simulink model "8Bit_MUX"  (R2019b)
settings: Solver=VariableStepAuto  StartTime=0.0  StopTime=10.0  RelTol=1e-3
libraries: hdlsllib x49
settings Model: Creator=cohen  LastModifiedBy=cohen

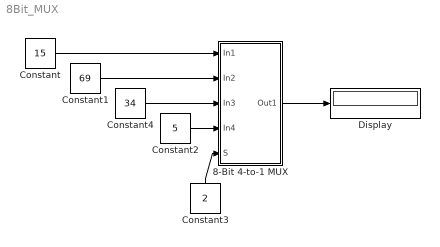
== system 8Bit_MUX ==
  8-Bit 4-to-1 MUX : Subsystem
  Constant : Constant  Value=15  OutDataTypeStr=uint8
  Constant1 : Constant  Value=69  OutDataTypeStr=uint8
  Constant2 : Constant  Value=5  OutDataTypeStr=uint8
  Constant3 : Constant  Value=2  OutDataTypeStr=uint8
  Constant4 : Constant  Value=34  OutDataTypeStr=uint8
  Display : Display
  wires:
  8-Bit 4-to-1 MUX/1(Out1) -> Display/1
  Constant/1 -> 8-Bit 4-to-1 MUX/1(In1)
  Constant1/1 -> 8-Bit 4-to-1 MUX/2(In2)
  Constant4/1 -> 8-Bit 4-to-1 MUX/3(In3)
  Constant2/1 -> 8-Bit 4-to-1 MUX/4(In4)
  Constant3/1 -> 8-Bit 4-to-1 MUX/5(S)

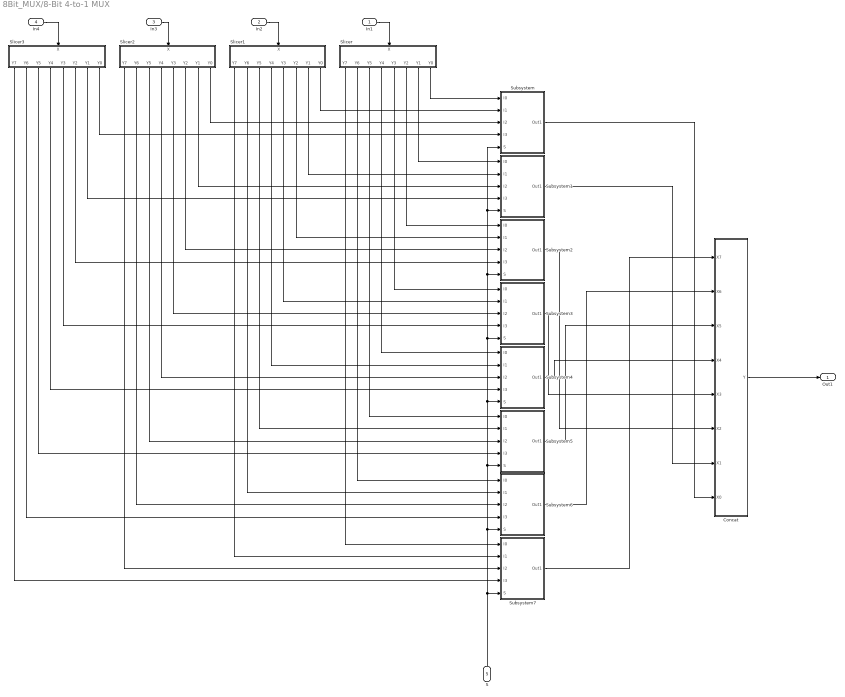
== system 8Bit_MUX/8-Bit 4-to-1 MUX ==
  In1 : Inport  OutDataTypeStr=uint8
  In2 : Inport  Port=2  OutDataTypeStr=uint8
  In3 : Inport  Port=3  OutDataTypeStr=uint8
  In4 : Inport  Port=4  OutDataTypeStr=uint8
  S : Inport  Port=5  OutDataTypeStr=uint8
  Concat : Subsystem
  Slicer : Subsystem
  Slicer1 : Subsystem
  Slicer2 : Subsystem
  Slicer3 : Subsystem
  Subsystem : Subsystem
  Subsystem1 : Subsystem
  Subsystem2 : Subsystem
  Subsystem3 : Subsystem
  Subsystem4 : Subsystem
  Subsystem5 : Subsystem
  Subsystem6 : Subsystem
  Subsystem7 : Subsystem
  Out1 : Outport  OutDataTypeStr=uint8
  wires:
  Slicer1/8(Y0) -> Subsystem/2(I1)
  Subsystem3/1(Out1) -> Concat/5(X3)
  Slicer/6(Y2) -> Subsystem2/1(I0)
  Slicer2/7(Y1) -> Subsystem1/3(I2)
  Subsystem2/1(Out1) -> Concat/6(X2)
  Concat/1(Y) -> Out1/1
  S/1 -> Subsystem7/5(S), Subsystem4/5(S), Subsystem1/5(S), Subsystem/5(S), Subsystem2/5(S), Subsystem3/5(S), Subsystem5/5(S), Subsystem6/5(S)
  Subsystem6/1(Out1) -> Concat/2(X6)
  Slicer2/3(Y5) -> Subsystem5/3(I2)
  Slicer3/4(Y4) -> Subsystem4/4(I3)
  Slicer2/2(Y6) -> Subsystem6/3(I2)
  Slicer/2(Y6) -> Subsystem6/1(I0)
  In2/1 -> Slicer1/1(X)
  Slicer2/1(Y7) -> Subsystem7/3(I2)
  Slicer3/7(Y1) -> Subsystem1/4(I3)
  Slicer/5(Y3) -> Subsystem3/1(I0)
  Slicer3/6(Y2) -> Subsystem2/4(I3)
  In1/1 -> Slicer/1(X)
  Slicer1/1(Y7) -> Subsystem7/2(I1)
  In3/1 -> Slicer2/1(X)
  Slicer/8(Y0) -> Subsystem/1(I0)
  Slicer1/4(Y4) -> Subsystem4/2(I1)
  Slicer2/4(Y4) -> Subsystem4/3(I2)
  Slicer1/3(Y5) -> Subsystem5/2(I1)
  Slicer3/5(Y3) -> Subsystem3/4(I3)
  Slicer/4(Y4) -> Subsystem4/1(I0)
  Slicer2/8(Y0) -> Subsystem/3(I2)
  Slicer1/5(Y3) -> Subsystem3/2(I1)
  Slicer1/7(Y1) -> Subsystem1/2(I1)
  Subsystem7/1(Out1) -> Concat/1(X7)
  Slicer1/6(Y2) -> Subsystem2/2(I1)
  Subsystem/1(Out1) -> Concat/8(X0)
  Subsystem4/1(Out1) -> Concat/4(X4)
  Subsystem5/1(Out1) -> Concat/3(X5)
  Slicer1/2(Y6) -> Subsystem6/2(I1)
  Slicer3/8(Y0) -> Subsystem/4(I3)
  Slicer2/6(Y2) -> Subsystem2/3(I2)
  Slicer/3(Y5) -> Subsystem5/1(I0)
  Slicer3/3(Y5) -> Subsystem5/4(I3)
  Slicer3/2(Y6) -> Subsystem6/4(I3)
  Slicer3/1(Y7) -> Subsystem7/4(I3)
  Slicer2/5(Y3) -> Subsystem3/3(I2)
  In4/1 -> Slicer3/1(X)
  Subsystem1/1(Out1) -> Concat/7(X1)
  Slicer/1(Y7) -> Subsystem7/1(I0)
  Slicer/7(Y1) -> Subsystem1/1(I0)

== system 8Bit_MUX/8-Bit 4-to-1 MUX/Concat ==
  X7 : Inport  OutDataTypeStr=boolean  SampleTime=1
  X6 : Inport  Port=2  OutDataTypeStr=boolean  SampleTime=1
  X5 : Inport  Port=3  OutDataTypeStr=boolean  SampleTime=1
  X4 : Inport  Port=4  OutDataTypeStr=boolean  SampleTime=1
  X3 : Inport  Port=5  OutDataTypeStr=boolean  SampleTime=1
  X2 : Inport  Port=6  OutDataTypeStr=boolean  SampleTime=1
  X1 : Inport  Port=7  OutDataTypeStr=boolean  SampleTime=1
  X0 : Inport  Port=8  OutDataTypeStr=boolean  SampleTime=1
  Bit Concat : hdlsllib/Logic and Bit Operations/Bit Concat  numInputs=8
      settings: SourceProductName=Simulink
  Y : Outport  SampleTime=1
  wires:
  X6/1 -> Bit Concat/2
  X2/1 -> Bit Concat/6
  X7/1 -> Bit Concat/1
  X0/1 -> Bit Concat/8
  Bit Concat/1 -> Y/1
  X3/1 -> Bit Concat/5
  X1/1 -> Bit Concat/7
  X5/1 -> Bit Concat/3
  X4/1 -> Bit Concat/4

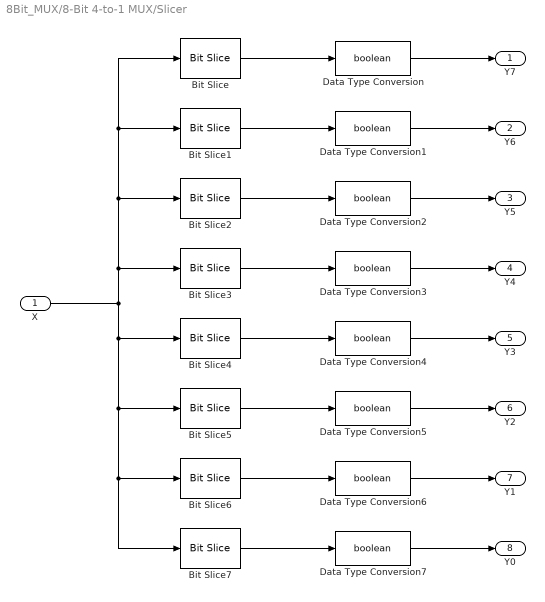
== system 8Bit_MUX/8-Bit 4-to-1 MUX/Slicer ==
  X : Inport  OutDataTypeStr=uint8  SampleTime=1
  Bit Slice : hdlsllib/Logic and Bit Operations/Bit Slice  lidx=7  ridx=7
      settings: SourceProductName=Simulink  SourceProductBaseCode=SL
  Bit Slice1 : hdlsllib/Logic and Bit Operations/Bit Slice  lidx=6  ridx=6
      settings: SourceProductName=Simulink  SourceProductBaseCode=SL
  Bit Slice2 : hdlsllib/Logic and Bit Operations/Bit Slice  lidx=5  ridx=5
      settings: SourceProductName=Simulink  SourceProductBaseCode=SL
  Bit Slice3 : hdlsllib/Logic and Bit Operations/Bit Slice  lidx=4  ridx=4
      settings: SourceProductName=Simulink  SourceProductBaseCode=SL
  Bit Slice4 : hdlsllib/Logic and Bit Operations/Bit Slice  lidx=3  ridx=3
      settings: SourceProductName=Simulink  SourceProductBaseCode=SL
  Bit Slice5 : hdlsllib/Logic and Bit Operations/Bit Slice  lidx=2  ridx=2
      settings: SourceProductName=Simulink  SourceProductBaseCode=SL
  Bit Slice6 : hdlsllib/Logic and Bit Operations/Bit Slice  lidx=1  ridx=1
      settings: SourceProductName=Simulink  SourceProductBaseCode=SL
  Bit Slice7 : hdlsllib/Logic and Bit Operations/Bit Slice  lidx=0  ridx=0
      settings: SourceProductName=Simulink  SourceProductBaseCode=SL
  Data Type Conversion{,1..7} (8 alike) : DataTypeConversion  OutDataTypeStr=boolean
  Y7 : Outport  OutDataTypeStr=boolean  SampleTime=1
  Y6 : Outport  Port=2  OutDataTypeStr=boolean  SampleTime=1
  Y5 : Outport  Port=3  OutDataTypeStr=boolean  SampleTime=1
  Y4 : Outport  Port=4  OutDataTypeStr=boolean
  Y3 : Outport  Port=5  OutDataTypeStr=boolean  SampleTime=1
  Y2 : Outport  Port=6  OutDataTypeStr=boolean  SampleTime=1
  Y1 : Outport  Port=7  OutDataTypeStr=boolean  SampleTime=1
  Y0 : Outport  Port=8  OutDataTypeStr=boolean  SampleTime=1
  wires:
  Bit Slice6/1 -> Data Type Conversion6/1
  X/1 -> Bit Slice3/1, Bit Slice2/1, Bit Slice1/1, Bit Slice/1, Bit Slice4/1, Bit Slice5/1, Bit Slice6/1, Bit Slice7/1
  Bit Slice/1 -> Data Type Conversion/1
  Bit Slice7/1 -> Data Type Conversion7/1
  Bit Slice4/1 -> Data Type Conversion4/1
  Bit Slice1/1 -> Data Type Conversion1/1
  Bit Slice3/1 -> Data Type Conversion3/1
  Data Type Conversion1/1 -> Y6/1
  Data Type Conversion7/1 -> Y0/1
  Data Type Conversion5/1 -> Y2/1
  Data Type Conversion3/1 -> Y4/1
  Data Type Conversion4/1 -> Y3/1
  Bit Slice2/1 -> Data Type Conversion2/1
  Bit Slice5/1 -> Data Type Conversion5/1
  Data Type Conversion6/1 -> Y1/1
  Data Type Conversion/1 -> Y7/1
  Data Type Conversion2/1 -> Y5/1

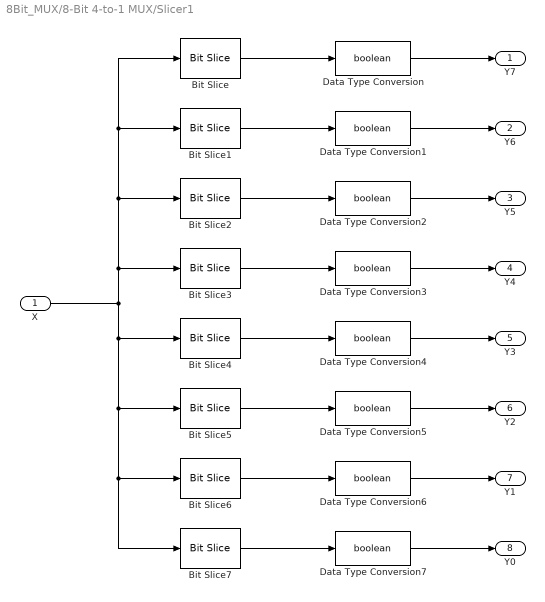
== system 8Bit_MUX/8-Bit 4-to-1 MUX/Slicer1 ==
  X : Inport  OutDataTypeStr=uint8  SampleTime=1
  Bit Slice : hdlsllib/Logic and Bit Operations/Bit Slice  lidx=7  ridx=7
      settings: SourceProductName=Simulink  SourceProductBaseCode=SL
  Bit Slice1 : hdlsllib/Logic and Bit Operations/Bit Slice  lidx=6  ridx=6
      settings: SourceProductName=Simulink  SourceProductBaseCode=SL
  Bit Slice2 : hdlsllib/Logic and Bit Operations/Bit Slice  lidx=5  ridx=5
      settings: SourceProductName=Simulink  SourceProductBaseCode=SL
  Bit Slice3 : hdlsllib/Logic and Bit Operations/Bit Slice  lidx=4  ridx=4
      settings: SourceProductName=Simulink  SourceProductBaseCode=SL
  Bit Slice4 : hdlsllib/Logic and Bit Operations/Bit Slice  lidx=3  ridx=3
      settings: SourceProductName=Simulink  SourceProductBaseCode=SL
  Bit Slice5 : hdlsllib/Logic and Bit Operations/Bit Slice  lidx=2  ridx=2
      settings: SourceProductName=Simulink  SourceProductBaseCode=SL
  Bit Slice6 : hdlsllib/Logic and Bit Operations/Bit Slice  lidx=1  ridx=1
      settings: SourceProductName=Simulink  SourceProductBaseCode=SL
  Bit Slice7 : hdlsllib/Logic and Bit Operations/Bit Slice  lidx=0  ridx=0
      settings: SourceProductName=Simulink  SourceProductBaseCode=SL
  Data Type Conversion{,1..7} (8 alike) : DataTypeConversion  OutDataTypeStr=boolean
  Y7 : Outport  OutDataTypeStr=boolean  SampleTime=1
  Y6 : Outport  Port=2  OutDataTypeStr=boolean  SampleTime=1
  Y5 : Outport  Port=3  OutDataTypeStr=boolean  SampleTime=1
  Y4 : Outport  Port=4  OutDataTypeStr=boolean
  Y3 : Outport  Port=5  OutDataTypeStr=boolean  SampleTime=1
  Y2 : Outport  Port=6  OutDataTypeStr=boolean  SampleTime=1
  Y1 : Outport  Port=7  OutDataTypeStr=boolean  SampleTime=1
  Y0 : Outport  Port=8  OutDataTypeStr=boolean  SampleTime=1
  wires:
  Bit Slice6/1 -> Data Type Conversion6/1
  X/1 -> Bit Slice3/1, Bit Slice2/1, Bit Slice1/1, Bit Slice/1, Bit Slice4/1, Bit Slice5/1, Bit Slice6/1, Bit Slice7/1
  Bit Slice/1 -> Data Type Conversion/1
  Bit Slice7/1 -> Data Type Conversion7/1
  Bit Slice4/1 -> Data Type Conversion4/1
  Bit Slice1/1 -> Data Type Conversion1/1
  Bit Slice3/1 -> Data Type Conversion3/1
  Data Type Conversion1/1 -> Y6/1
  Data Type Conversion7/1 -> Y0/1
  Data Type Conversion5/1 -> Y2/1
  Data Type Conversion3/1 -> Y4/1
  Data Type Conversion4/1 -> Y3/1
  Bit Slice2/1 -> Data Type Conversion2/1
  Bit Slice5/1 -> Data Type Conversion5/1
  Data Type Conversion6/1 -> Y1/1
  Data Type Conversion/1 -> Y7/1
  Data Type Conversion2/1 -> Y5/1

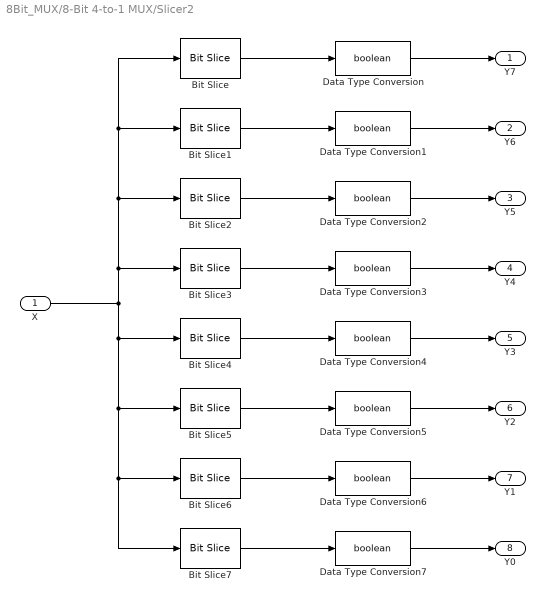
== system 8Bit_MUX/8-Bit 4-to-1 MUX/Slicer2 ==
  X : Inport  OutDataTypeStr=uint8  SampleTime=1
  Bit Slice : hdlsllib/Logic and Bit Operations/Bit Slice  lidx=7  ridx=7
      settings: SourceProductName=Simulink  SourceProductBaseCode=SL
  Bit Slice1 : hdlsllib/Logic and Bit Operations/Bit Slice  lidx=6  ridx=6
      settings: SourceProductName=Simulink  SourceProductBaseCode=SL
  Bit Slice2 : hdlsllib/Logic and Bit Operations/Bit Slice  lidx=5  ridx=5
      settings: SourceProductName=Simulink  SourceProductBaseCode=SL
  Bit Slice3 : hdlsllib/Logic and Bit Operations/Bit Slice  lidx=4  ridx=4
      settings: SourceProductName=Simulink  SourceProductBaseCode=SL
  Bit Slice4 : hdlsllib/Logic and Bit Operations/Bit Slice  lidx=3  ridx=3
      settings: SourceProductName=Simulink  SourceProductBaseCode=SL
  Bit Slice5 : hdlsllib/Logic and Bit Operations/Bit Slice  lidx=2  ridx=2
      settings: SourceProductName=Simulink  SourceProductBaseCode=SL
  Bit Slice6 : hdlsllib/Logic and Bit Operations/Bit Slice  lidx=1  ridx=1
      settings: SourceProductName=Simulink  SourceProductBaseCode=SL
  Bit Slice7 : hdlsllib/Logic and Bit Operations/Bit Slice  lidx=0  ridx=0
      settings: SourceProductName=Simulink  SourceProductBaseCode=SL
  Data Type Conversion{,1..7} (8 alike) : DataTypeConversion  OutDataTypeStr=boolean
  Y7 : Outport  OutDataTypeStr=boolean  SampleTime=1
  Y6 : Outport  Port=2  OutDataTypeStr=boolean  SampleTime=1
  Y5 : Outport  Port=3  OutDataTypeStr=boolean  SampleTime=1
  Y4 : Outport  Port=4  OutDataTypeStr=boolean
  Y3 : Outport  Port=5  OutDataTypeStr=boolean  SampleTime=1
  Y2 : Outport  Port=6  OutDataTypeStr=boolean  SampleTime=1
  Y1 : Outport  Port=7  OutDataTypeStr=boolean  SampleTime=1
  Y0 : Outport  Port=8  OutDataTypeStr=boolean  SampleTime=1
  wires:
  Bit Slice6/1 -> Data Type Conversion6/1
  X/1 -> Bit Slice3/1, Bit Slice2/1, Bit Slice1/1, Bit Slice/1, Bit Slice4/1, Bit Slice5/1, Bit Slice6/1, Bit Slice7/1
  Bit Slice/1 -> Data Type Conversion/1
  Bit Slice7/1 -> Data Type Conversion7/1
  Bit Slice4/1 -> Data Type Conversion4/1
  Bit Slice1/1 -> Data Type Conversion1/1
  Bit Slice3/1 -> Data Type Conversion3/1
  Data Type Conversion1/1 -> Y6/1
  Data Type Conversion7/1 -> Y0/1
  Data Type Conversion5/1 -> Y2/1
  Data Type Conversion3/1 -> Y4/1
  Data Type Conversion4/1 -> Y3/1
  Bit Slice2/1 -> Data Type Conversion2/1
  Bit Slice5/1 -> Data Type Conversion5/1
  Data Type Conversion6/1 -> Y1/1
  Data Type Conversion/1 -> Y7/1
  Data Type Conversion2/1 -> Y5/1

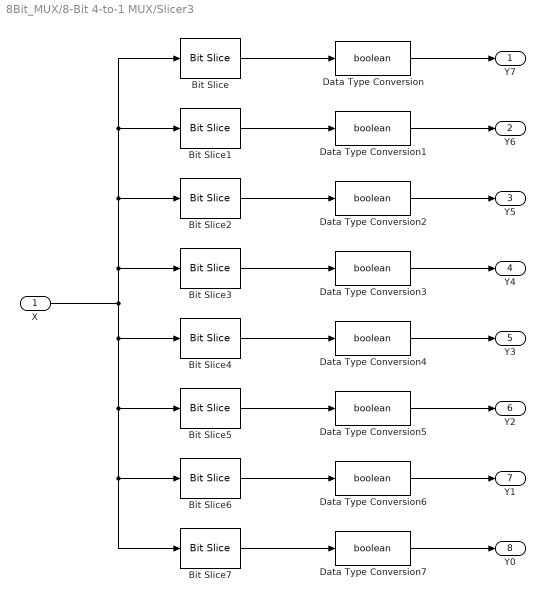
== system 8Bit_MUX/8-Bit 4-to-1 MUX/Slicer3 ==
  X : Inport  OutDataTypeStr=uint8  SampleTime=1
  Bit Slice : hdlsllib/Logic and Bit Operations/Bit Slice  lidx=7  ridx=7
      settings: SourceProductName=Simulink  SourceProductBaseCode=SL
  Bit Slice1 : hdlsllib/Logic and Bit Operations/Bit Slice  lidx=6  ridx=6
      settings: SourceProductName=Simulink  SourceProductBaseCode=SL
  Bit Slice2 : hdlsllib/Logic and Bit Operations/Bit Slice  lidx=5  ridx=5
      settings: SourceProductName=Simulink  SourceProductBaseCode=SL
  Bit Slice3 : hdlsllib/Logic and Bit Operations/Bit Slice  lidx=4  ridx=4
      settings: SourceProductName=Simulink  SourceProductBaseCode=SL
  Bit Slice4 : hdlsllib/Logic and Bit Operations/Bit Slice  lidx=3  ridx=3
      settings: SourceProductName=Simulink  SourceProductBaseCode=SL
  Bit Slice5 : hdlsllib/Logic and Bit Operations/Bit Slice  lidx=2  ridx=2
      settings: SourceProductName=Simulink  SourceProductBaseCode=SL
  Bit Slice6 : hdlsllib/Logic and Bit Operations/Bit Slice  lidx=1  ridx=1
      settings: SourceProductName=Simulink  SourceProductBaseCode=SL
  Bit Slice7 : hdlsllib/Logic and Bit Operations/Bit Slice  lidx=0  ridx=0
      settings: SourceProductName=Simulink  SourceProductBaseCode=SL
  Data Type Conversion{,1..7} (8 alike) : DataTypeConversion  OutDataTypeStr=boolean
  Y7 : Outport  OutDataTypeStr=boolean  SampleTime=1
  Y6 : Outport  Port=2  OutDataTypeStr=boolean  SampleTime=1
  Y5 : Outport  Port=3  OutDataTypeStr=boolean  SampleTime=1
  Y4 : Outport  Port=4  OutDataTypeStr=boolean
  Y3 : Outport  Port=5  OutDataTypeStr=boolean  SampleTime=1
  Y2 : Outport  Port=6  OutDataTypeStr=boolean  SampleTime=1
  Y1 : Outport  Port=7  OutDataTypeStr=boolean  SampleTime=1
  Y0 : Outport  Port=8  OutDataTypeStr=boolean  SampleTime=1
  wires:
  Bit Slice6/1 -> Data Type Conversion6/1
  X/1 -> Bit Slice3/1, Bit Slice2/1, Bit Slice1/1, Bit Slice/1, Bit Slice4/1, Bit Slice5/1, Bit Slice6/1, Bit Slice7/1
  Bit Slice/1 -> Data Type Conversion/1
  Bit Slice7/1 -> Data Type Conversion7/1
  Bit Slice4/1 -> Data Type Conversion4/1
  Bit Slice1/1 -> Data Type Conversion1/1
  Bit Slice3/1 -> Data Type Conversion3/1
  Data Type Conversion1/1 -> Y6/1
  Data Type Conversion7/1 -> Y0/1
  Data Type Conversion5/1 -> Y2/1
  Data Type Conversion3/1 -> Y4/1
  Data Type Conversion4/1 -> Y3/1
  Bit Slice2/1 -> Data Type Conversion2/1
  Bit Slice5/1 -> Data Type Conversion5/1
  Data Type Conversion6/1 -> Y1/1
  Data Type Conversion/1 -> Y7/1
  Data Type Conversion2/1 -> Y5/1

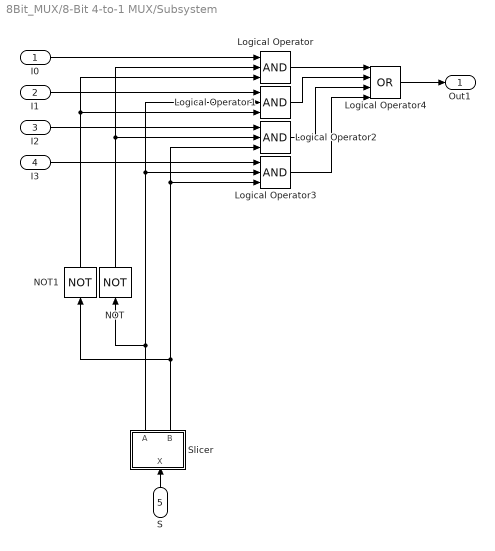
== system 8Bit_MUX/8-Bit 4-to-1 MUX/Subsystem ==
  I0 : Inport  OutDataTypeStr=boolean
  I1 : Inport  Port=2  OutDataTypeStr=boolean
  I2 : Inport  Port=3  OutDataTypeStr=boolean
  I3 : Inport  Port=4  OutDataTypeStr=boolean
  S : Inport  Port=5  OutDataTypeStr=uint8
  Logical Operator{,1..3} (4 alike) : Logic  Inputs=3  AllPortsSameDT=off  OutDataTypeStr=boolean
  Logical Operator4 : Logic  Operator=OR  Inputs=4  AllPortsSameDT=off  OutDataTypeStr=boolean
  NOT : Logic  Operator=NOT  IconShape=distinctive  AllPortsSameDT=off  OutDataTypeStr=boolean
  NOT1 : Logic  Operator=NOT  IconShape=distinctive  AllPortsSameDT=off  OutDataTypeStr=boolean
  Slicer : Subsystem
  Out1 : Outport  OutDataTypeStr=boolean
  wires:
  Logical Operator1/1 -> Logical Operator4/2
  NOT/1 -> Logical Operator/2, Logical Operator2/2
  I1/1 -> Logical Operator1/1
  I2/1 -> Logical Operator2/1
  NOT1/1 -> Logical Operator/3, Logical Operator1/3
  I3/1 -> Logical Operator3/1
  I0/1 -> Logical Operator/1
  Logical Operator2/1 -> Logical Operator4/3
  Logical Operator4/1 -> Out1/1
  Logical Operator3/1 -> Logical Operator4/4
  Logical Operator/1 -> Logical Operator4/1
  S/1 -> Slicer/1(X)
  Slicer/2(B) -> NOT1/1, Logical Operator2/3, Logical Operator3/3
  Slicer/1(A) -> NOT/1, Logical Operator1/2, Logical Operator3/2

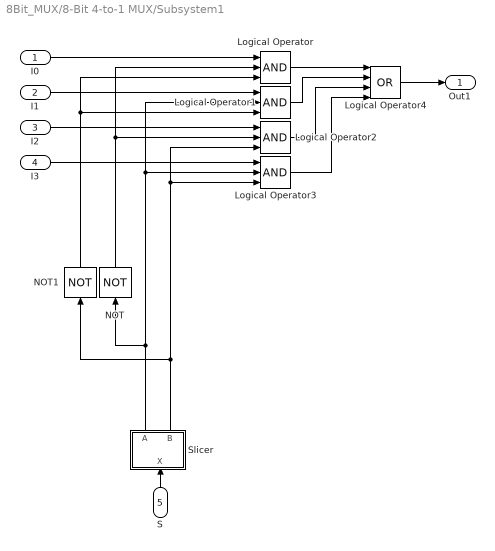
== system 8Bit_MUX/8-Bit 4-to-1 MUX/Subsystem1 ==
  I0 : Inport  OutDataTypeStr=boolean
  I1 : Inport  Port=2  OutDataTypeStr=boolean
  I2 : Inport  Port=3  OutDataTypeStr=boolean
  I3 : Inport  Port=4  OutDataTypeStr=boolean
  S : Inport  Port=5  OutDataTypeStr=uint8
  Logical Operator{,1..3} (4 alike) : Logic  Inputs=3  AllPortsSameDT=off  OutDataTypeStr=boolean
  Logical Operator4 : Logic  Operator=OR  Inputs=4  AllPortsSameDT=off  OutDataTypeStr=boolean
  NOT : Logic  Operator=NOT  IconShape=distinctive  AllPortsSameDT=off  OutDataTypeStr=boolean
  NOT1 : Logic  Operator=NOT  IconShape=distinctive  AllPortsSameDT=off  OutDataTypeStr=boolean
  Slicer : Subsystem
  Out1 : Outport  OutDataTypeStr=boolean
  wires:
  Logical Operator1/1 -> Logical Operator4/2
  NOT/1 -> Logical Operator/2, Logical Operator2/2
  I1/1 -> Logical Operator1/1
  I2/1 -> Logical Operator2/1
  NOT1/1 -> Logical Operator/3, Logical Operator1/3
  I3/1 -> Logical Operator3/1
  I0/1 -> Logical Operator/1
  Logical Operator2/1 -> Logical Operator4/3
  Logical Operator4/1 -> Out1/1
  Logical Operator3/1 -> Logical Operator4/4
  Logical Operator/1 -> Logical Operator4/1
  S/1 -> Slicer/1(X)
  Slicer/2(B) -> NOT1/1, Logical Operator2/3, Logical Operator3/3
  Slicer/1(A) -> NOT/1, Logical Operator1/2, Logical Operator3/2

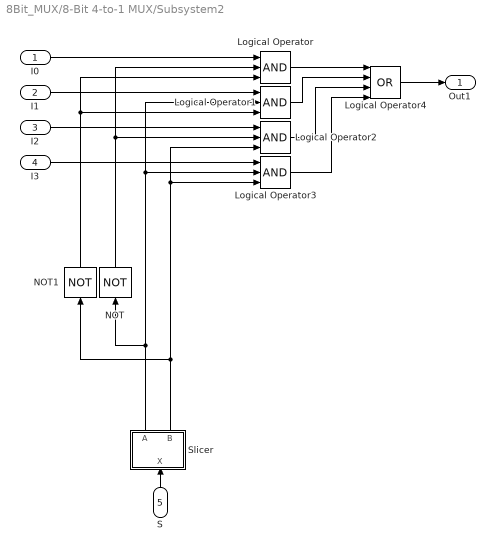
== system 8Bit_MUX/8-Bit 4-to-1 MUX/Subsystem2 ==
  I0 : Inport  OutDataTypeStr=boolean
  I1 : Inport  Port=2  OutDataTypeStr=boolean
  I2 : Inport  Port=3  OutDataTypeStr=boolean
  I3 : Inport  Port=4  OutDataTypeStr=boolean
  S : Inport  Port=5  OutDataTypeStr=uint8
  Logical Operator{,1..3} (4 alike) : Logic  Inputs=3  AllPortsSameDT=off  OutDataTypeStr=boolean
  Logical Operator4 : Logic  Operator=OR  Inputs=4  AllPortsSameDT=off  OutDataTypeStr=boolean
  NOT : Logic  Operator=NOT  IconShape=distinctive  AllPortsSameDT=off  OutDataTypeStr=boolean
  NOT1 : Logic  Operator=NOT  IconShape=distinctive  AllPortsSameDT=off  OutDataTypeStr=boolean
  Slicer : Subsystem
  Out1 : Outport  OutDataTypeStr=boolean
  wires:
  Logical Operator1/1 -> Logical Operator4/2
  NOT/1 -> Logical Operator/2, Logical Operator2/2
  I1/1 -> Logical Operator1/1
  I2/1 -> Logical Operator2/1
  NOT1/1 -> Logical Operator/3, Logical Operator1/3
  I3/1 -> Logical Operator3/1
  I0/1 -> Logical Operator/1
  Logical Operator2/1 -> Logical Operator4/3
  Logical Operator4/1 -> Out1/1
  Logical Operator3/1 -> Logical Operator4/4
  Logical Operator/1 -> Logical Operator4/1
  S/1 -> Slicer/1(X)
  Slicer/2(B) -> NOT1/1, Logical Operator2/3, Logical Operator3/3
  Slicer/1(A) -> NOT/1, Logical Operator1/2, Logical Operator3/2

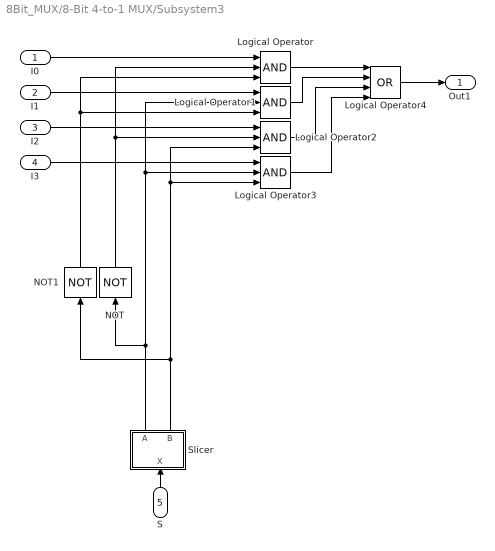
== system 8Bit_MUX/8-Bit 4-to-1 MUX/Subsystem3 ==
  I0 : Inport  OutDataTypeStr=boolean
  I1 : Inport  Port=2  OutDataTypeStr=boolean
  I2 : Inport  Port=3  OutDataTypeStr=boolean
  I3 : Inport  Port=4  OutDataTypeStr=boolean
  S : Inport  Port=5  OutDataTypeStr=uint8
  Logical Operator{,1..3} (4 alike) : Logic  Inputs=3  AllPortsSameDT=off  OutDataTypeStr=boolean
  Logical Operator4 : Logic  Operator=OR  Inputs=4  AllPortsSameDT=off  OutDataTypeStr=boolean
  NOT : Logic  Operator=NOT  IconShape=distinctive  AllPortsSameDT=off  OutDataTypeStr=boolean
  NOT1 : Logic  Operator=NOT  IconShape=distinctive  AllPortsSameDT=off  OutDataTypeStr=boolean
  Slicer : Subsystem
  Out1 : Outport  OutDataTypeStr=boolean
  wires:
  Logical Operator1/1 -> Logical Operator4/2
  NOT/1 -> Logical Operator/2, Logical Operator2/2
  I1/1 -> Logical Operator1/1
  I2/1 -> Logical Operator2/1
  NOT1/1 -> Logical Operator/3, Logical Operator1/3
  I3/1 -> Logical Operator3/1
  I0/1 -> Logical Operator/1
  Logical Operator2/1 -> Logical Operator4/3
  Logical Operator4/1 -> Out1/1
  Logical Operator3/1 -> Logical Operator4/4
  Logical Operator/1 -> Logical Operator4/1
  S/1 -> Slicer/1(X)
  Slicer/2(B) -> NOT1/1, Logical Operator2/3, Logical Operator3/3
  Slicer/1(A) -> NOT/1, Logical Operator1/2, Logical Operator3/2

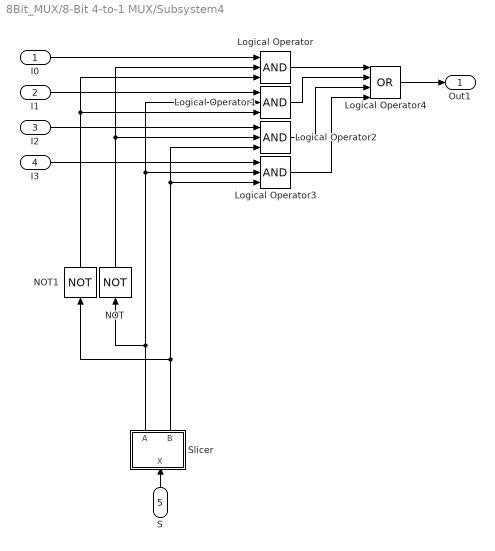
== system 8Bit_MUX/8-Bit 4-to-1 MUX/Subsystem4 ==
  I0 : Inport  OutDataTypeStr=boolean
  I1 : Inport  Port=2  OutDataTypeStr=boolean
  I2 : Inport  Port=3  OutDataTypeStr=boolean
  I3 : Inport  Port=4  OutDataTypeStr=boolean
  S : Inport  Port=5  OutDataTypeStr=uint8
  Logical Operator{,1..3} (4 alike) : Logic  Inputs=3  AllPortsSameDT=off  OutDataTypeStr=boolean
  Logical Operator4 : Logic  Operator=OR  Inputs=4  AllPortsSameDT=off  OutDataTypeStr=boolean
  NOT : Logic  Operator=NOT  IconShape=distinctive  AllPortsSameDT=off  OutDataTypeStr=boolean
  NOT1 : Logic  Operator=NOT  IconShape=distinctive  AllPortsSameDT=off  OutDataTypeStr=boolean
  Slicer : Subsystem
  Out1 : Outport  OutDataTypeStr=boolean
  wires:
  Logical Operator1/1 -> Logical Operator4/2
  NOT/1 -> Logical Operator/2, Logical Operator2/2
  I1/1 -> Logical Operator1/1
  I2/1 -> Logical Operator2/1
  NOT1/1 -> Logical Operator/3, Logical Operator1/3
  I3/1 -> Logical Operator3/1
  I0/1 -> Logical Operator/1
  Logical Operator2/1 -> Logical Operator4/3
  Logical Operator4/1 -> Out1/1
  Logical Operator3/1 -> Logical Operator4/4
  Logical Operator/1 -> Logical Operator4/1
  S/1 -> Slicer/1(X)
  Slicer/2(B) -> NOT1/1, Logical Operator2/3, Logical Operator3/3
  Slicer/1(A) -> NOT/1, Logical Operator1/2, Logical Operator3/2

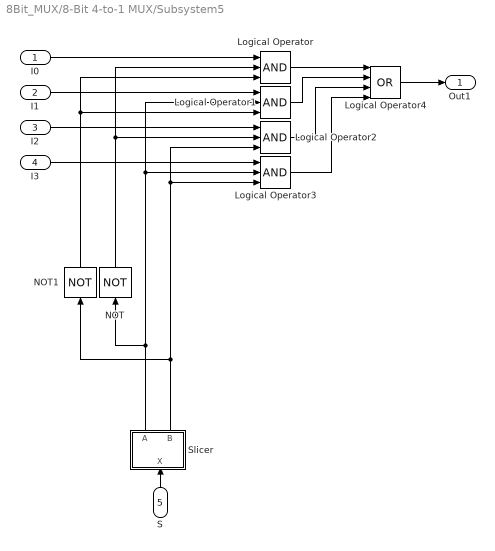
== system 8Bit_MUX/8-Bit 4-to-1 MUX/Subsystem5 ==
  I0 : Inport  OutDataTypeStr=boolean
  I1 : Inport  Port=2  OutDataTypeStr=boolean
  I2 : Inport  Port=3  OutDataTypeStr=boolean
  I3 : Inport  Port=4  OutDataTypeStr=boolean
  S : Inport  Port=5  OutDataTypeStr=uint8
  Logical Operator{,1..3} (4 alike) : Logic  Inputs=3  AllPortsSameDT=off  OutDataTypeStr=boolean
  Logical Operator4 : Logic  Operator=OR  Inputs=4  AllPortsSameDT=off  OutDataTypeStr=boolean
  NOT : Logic  Operator=NOT  IconShape=distinctive  AllPortsSameDT=off  OutDataTypeStr=boolean
  NOT1 : Logic  Operator=NOT  IconShape=distinctive  AllPortsSameDT=off  OutDataTypeStr=boolean
  Slicer : Subsystem
  Out1 : Outport  OutDataTypeStr=boolean
  wires:
  Logical Operator1/1 -> Logical Operator4/2
  NOT/1 -> Logical Operator/2, Logical Operator2/2
  I1/1 -> Logical Operator1/1
  I2/1 -> Logical Operator2/1
  NOT1/1 -> Logical Operator/3, Logical Operator1/3
  I3/1 -> Logical Operator3/1
  I0/1 -> Logical Operator/1
  Logical Operator2/1 -> Logical Operator4/3
  Logical Operator4/1 -> Out1/1
  Logical Operator3/1 -> Logical Operator4/4
  Logical Operator/1 -> Logical Operator4/1
  S/1 -> Slicer/1(X)
  Slicer/2(B) -> NOT1/1, Logical Operator2/3, Logical Operator3/3
  Slicer/1(A) -> NOT/1, Logical Operator1/2, Logical Operator3/2

== system 8Bit_MUX/8-Bit 4-to-1 MUX/Subsystem6 ==
  I0 : Inport  OutDataTypeStr=boolean
  I1 : Inport  Port=2  OutDataTypeStr=boolean
  I2 : Inport  Port=3  OutDataTypeStr=boolean
  I3 : Inport  Port=4  OutDataTypeStr=boolean
  S : Inport  Port=5  OutDataTypeStr=uint8
  Logical Operator{,1..3} (4 alike) : Logic  Inputs=3  AllPortsSameDT=off  OutDataTypeStr=boolean
  Logical Operator4 : Logic  Operator=OR  Inputs=4  AllPortsSameDT=off  OutDataTypeStr=boolean
  NOT : Logic  Operator=NOT  IconShape=distinctive  AllPortsSameDT=off  OutDataTypeStr=boolean
  NOT1 : Logic  Operator=NOT  IconShape=distinctive  AllPortsSameDT=off  OutDataTypeStr=boolean
  Slicer : Subsystem
  Out1 : Outport  OutDataTypeStr=boolean
  wires:
  Logical Operator1/1 -> Logical Operator4/2
  NOT/1 -> Logical Operator/2, Logical Operator2/2
  I1/1 -> Logical Operator1/1
  I2/1 -> Logical Operator2/1
  NOT1/1 -> Logical Operator/3, Logical Operator1/3
  I3/1 -> Logical Operator3/1
  I0/1 -> Logical Operator/1
  Logical Operator2/1 -> Logical Operator4/3
  Logical Operator4/1 -> Out1/1
  Logical Operator3/1 -> Logical Operator4/4
  Logical Operator/1 -> Logical Operator4/1
  S/1 -> Slicer/1(X)
  Slicer/2(B) -> NOT1/1, Logical Operator2/3, Logical Operator3/3
  Slicer/1(A) -> NOT/1, Logical Operator1/2, Logical Operator3/2

== system 8Bit_MUX/8-Bit 4-to-1 MUX/Subsystem7 ==
  I0 : Inport  OutDataTypeStr=boolean
  I1 : Inport  Port=2  OutDataTypeStr=boolean
  I2 : Inport  Port=3  OutDataTypeStr=boolean
  I3 : Inport  Port=4  OutDataTypeStr=boolean
  S : Inport  Port=5  OutDataTypeStr=uint8
  Logical Operator{,1..3} (4 alike) : Logic  Inputs=3  AllPortsSameDT=off  OutDataTypeStr=boolean
  Logical Operator4 : Logic  Operator=OR  Inputs=4  AllPortsSameDT=off  OutDataTypeStr=boolean
  NOT : Logic  Operator=NOT  IconShape=distinctive  AllPortsSameDT=off  OutDataTypeStr=boolean
  NOT1 : Logic  Operator=NOT  IconShape=distinctive  AllPortsSameDT=off  OutDataTypeStr=boolean
  Slicer : Subsystem
  Out1 : Outport  OutDataTypeStr=boolean
  wires:
  Logical Operator1/1 -> Logical Operator4/2
  NOT/1 -> Logical Operator/2, Logical Operator2/2
  I1/1 -> Logical Operator1/1
  I2/1 -> Logical Operator2/1
  NOT1/1 -> Logical Operator/3, Logical Operator1/3
  I3/1 -> Logical Operator3/1
  I0/1 -> Logical Operator/1
  Logical Operator2/1 -> Logical Operator4/3
  Logical Operator4/1 -> Out1/1
  Logical Operator3/1 -> Logical Operator4/4
  Logical Operator/1 -> Logical Operator4/1
  S/1 -> Slicer/1(X)
  Slicer/2(B) -> NOT1/1, Logical Operator2/3, Logical Operator3/3
  Slicer/1(A) -> NOT/1, Logical Operator1/2, Logical Operator3/2

== system 8Bit_MUX/8-Bit 4-to-1 MUX/Subsystem/Slicer ==
  X : Inport  OutDataTypeStr=uint8  SampleTime=1
  Bit Slice6 : hdlsllib/Logic and Bit Operations/Bit Slice  lidx=1  ridx=1
      settings: SourceProductName=Simulink  SourceProductBaseCode=SL
  Bit Slice7 : hdlsllib/Logic and Bit Operations/Bit Slice  lidx=0  ridx=0
      settings: SourceProductName=Simulink  SourceProductBaseCode=SL
  Data Type Conversion6 : DataTypeConversion  OutDataTypeStr=boolean
  Data Type Conversion7 : DataTypeConversion  OutDataTypeStr=boolean
  A : Outport  OutDataTypeStr=boolean  SampleTime=1
  B : Outport  Port=2  OutDataTypeStr=boolean  SampleTime=1
  wires:
  Bit Slice6/1 -> Data Type Conversion6/1
  X/1 -> Bit Slice6/1, Bit Slice7/1
  Bit Slice7/1 -> Data Type Conversion7/1
  Data Type Conversion7/1 -> A/1
  Data Type Conversion6/1 -> B/1

== system 8Bit_MUX/8-Bit 4-to-1 MUX/Subsystem1/Slicer ==
  X : Inport  OutDataTypeStr=uint8  SampleTime=1
  Bit Slice6 : hdlsllib/Logic and Bit Operations/Bit Slice  lidx=1  ridx=1
      settings: SourceProductName=Simulink  SourceProductBaseCode=SL
  Bit Slice7 : hdlsllib/Logic and Bit Operations/Bit Slice  lidx=0  ridx=0
      settings: SourceProductName=Simulink  SourceProductBaseCode=SL
  Data Type Conversion6 : DataTypeConversion  OutDataTypeStr=boolean
  Data Type Conversion7 : DataTypeConversion  OutDataTypeStr=boolean
  A : Outport  OutDataTypeStr=boolean  SampleTime=1
  B : Outport  Port=2  OutDataTypeStr=boolean  SampleTime=1
  wires:
  Bit Slice6/1 -> Data Type Conversion6/1
  X/1 -> Bit Slice6/1, Bit Slice7/1
  Bit Slice7/1 -> Data Type Conversion7/1
  Data Type Conversion7/1 -> A/1
  Data Type Conversion6/1 -> B/1

== system 8Bit_MUX/8-Bit 4-to-1 MUX/Subsystem2/Slicer ==
  X : Inport  OutDataTypeStr=uint8  SampleTime=1
  Bit Slice6 : hdlsllib/Logic and Bit Operations/Bit Slice  lidx=1  ridx=1
      settings: SourceProductName=Simulink  SourceProductBaseCode=SL
  Bit Slice7 : hdlsllib/Logic and Bit Operations/Bit Slice  lidx=0  ridx=0
      settings: SourceProductName=Simulink  SourceProductBaseCode=SL
  Data Type Conversion6 : DataTypeConversion  OutDataTypeStr=boolean
  Data Type Conversion7 : DataTypeConversion  OutDataTypeStr=boolean
  A : Outport  OutDataTypeStr=boolean  SampleTime=1
  B : Outport  Port=2  OutDataTypeStr=boolean  SampleTime=1
  wires:
  Bit Slice6/1 -> Data Type Conversion6/1
  X/1 -> Bit Slice6/1, Bit Slice7/1
  Bit Slice7/1 -> Data Type Conversion7/1
  Data Type Conversion7/1 -> A/1
  Data Type Conversion6/1 -> B/1

== system 8Bit_MUX/8-Bit 4-to-1 MUX/Subsystem3/Slicer ==
  X : Inport  OutDataTypeStr=uint8  SampleTime=1
  Bit Slice6 : hdlsllib/Logic and Bit Operations/Bit Slice  lidx=1  ridx=1
      settings: SourceProductName=Simulink  SourceProductBaseCode=SL
  Bit Slice7 : hdlsllib/Logic and Bit Operations/Bit Slice  lidx=0  ridx=0
      settings: SourceProductName=Simulink  SourceProductBaseCode=SL
  Data Type Conversion6 : DataTypeConversion  OutDataTypeStr=boolean
  Data Type Conversion7 : DataTypeConversion  OutDataTypeStr=boolean
  A : Outport  OutDataTypeStr=boolean  SampleTime=1
  B : Outport  Port=2  OutDataTypeStr=boolean  SampleTime=1
  wires:
  Bit Slice6/1 -> Data Type Conversion6/1
  X/1 -> Bit Slice6/1, Bit Slice7/1
  Bit Slice7/1 -> Data Type Conversion7/1
  Data Type Conversion7/1 -> A/1
  Data Type Conversion6/1 -> B/1

== system 8Bit_MUX/8-Bit 4-to-1 MUX/Subsystem4/Slicer ==
  X : Inport  OutDataTypeStr=uint8  SampleTime=1
  Bit Slice6 : hdlsllib/Logic and Bit Operations/Bit Slice  lidx=1  ridx=1
      settings: SourceProductName=Simulink  SourceProductBaseCode=SL
  Bit Slice7 : hdlsllib/Logic and Bit Operations/Bit Slice  lidx=0  ridx=0
      settings: SourceProductName=Simulink  SourceProductBaseCode=SL
  Data Type Conversion6 : DataTypeConversion  OutDataTypeStr=boolean
  Data Type Conversion7 : DataTypeConversion  OutDataTypeStr=boolean
  A : Outport  OutDataTypeStr=boolean  SampleTime=1
  B : Outport  Port=2  OutDataTypeStr=boolean  SampleTime=1
  wires:
  Bit Slice6/1 -> Data Type Conversion6/1
  X/1 -> Bit Slice6/1, Bit Slice7/1
  Bit Slice7/1 -> Data Type Conversion7/1
  Data Type Conversion7/1 -> A/1
  Data Type Conversion6/1 -> B/1

== system 8Bit_MUX/8-Bit 4-to-1 MUX/Subsystem5/Slicer ==
  X : Inport  OutDataTypeStr=uint8  SampleTime=1
  Bit Slice6 : hdlsllib/Logic and Bit Operations/Bit Slice  lidx=1  ridx=1
      settings: SourceProductName=Simulink  SourceProductBaseCode=SL
  Bit Slice7 : hdlsllib/Logic and Bit Operations/Bit Slice  lidx=0  ridx=0
      settings: SourceProductName=Simulink  SourceProductBaseCode=SL
  Data Type Conversion6 : DataTypeConversion  OutDataTypeStr=boolean
  Data Type Conversion7 : DataTypeConversion  OutDataTypeStr=boolean
  A : Outport  OutDataTypeStr=boolean  SampleTime=1
  B : Outport  Port=2  OutDataTypeStr=boolean  SampleTime=1
  wires:
  Bit Slice6/1 -> Data Type Conversion6/1
  X/1 -> Bit Slice6/1, Bit Slice7/1
  Bit Slice7/1 -> Data Type Conversion7/1
  Data Type Conversion7/1 -> A/1
  Data Type Conversion6/1 -> B/1

== system 8Bit_MUX/8-Bit 4-to-1 MUX/Subsystem6/Slicer ==
  X : Inport  OutDataTypeStr=uint8  SampleTime=1
  Bit Slice6 : hdlsllib/Logic and Bit Operations/Bit Slice  lidx=1  ridx=1
      settings: SourceProductName=Simulink  SourceProductBaseCode=SL
  Bit Slice7 : hdlsllib/Logic and Bit Operations/Bit Slice  lidx=0  ridx=0
      settings: SourceProductName=Simulink  SourceProductBaseCode=SL
  Data Type Conversion6 : DataTypeConversion  OutDataTypeStr=boolean
  Data Type Conversion7 : DataTypeConversion  OutDataTypeStr=boolean
  A : Outport  OutDataTypeStr=boolean  SampleTime=1
  B : Outport  Port=2  OutDataTypeStr=boolean  SampleTime=1
  wires:
  Bit Slice6/1 -> Data Type Conversion6/1
  X/1 -> Bit Slice6/1, Bit Slice7/1
  Bit Slice7/1 -> Data Type Conversion7/1
  Data Type Conversion7/1 -> A/1
  Data Type Conversion6/1 -> B/1

== system 8Bit_MUX/8-Bit 4-to-1 MUX/Subsystem7/Slicer ==
  X : Inport  OutDataTypeStr=uint8  SampleTime=1
  Bit Slice6 : hdlsllib/Logic and Bit Operations/Bit Slice  lidx=1  ridx=1
      settings: SourceProductName=Simulink  SourceProductBaseCode=SL
  Bit Slice7 : hdlsllib/Logic and Bit Operations/Bit Slice  lidx=0  ridx=0
      settings: SourceProductName=Simulink  SourceProductBaseCode=SL
  Data Type Conversion6 : DataTypeConversion  OutDataTypeStr=boolean
  Data Type Conversion7 : DataTypeConversion  OutDataTypeStr=boolean
  A : Outport  OutDataTypeStr=boolean  SampleTime=1
  B : Outport  Port=2  OutDataTypeStr=boolean  SampleTime=1
  wires:
  Bit Slice6/1 -> Data Type Conversion6/1
  X/1 -> Bit Slice6/1, Bit Slice7/1
  Bit Slice7/1 -> Data Type Conversion7/1
  Data Type Conversion7/1 -> A/1
  Data Type Conversion6/1 -> B/1
